simulink model "test"  (R2022b)
settings: Solver=VariableStepAuto  StartTime=0.0  StopTime=300  RelTol=1e-3
values from neighbouring files (symbols this model uses):
  m_pw = zeros(nvw,nwr)    [fun_getwindpowercurve_v4.m]
  pinitwindgen = 0.5161    [WGmodel_startup.m]    (also in WGmodel_startup_v2.m; WGmodel_startup_v3.m = pinitwindgen(1))
  R = 0.05    [WGmodel_startup.m]    (also in WGmodel_startup_v2.m; WGmodel_startup_v3.m)
  Tc2 = 0.05    [WGmodel_startup.m]    (also in WGmodel_startup_v2.m; WGmodel_startup_v3.m)
  v_beta = 0:1:2    [WGmodel_startup.m]    (also in fun_getwindpowercurve_v2.m = 0.5)
  v_pwdel = 0.9 * max(m_pw,[],2)    [fun_getwindpowercurve_v2.m]    (also in fun_getwindpowercurve_v3.m = (1-deload) * v_pwmpp; fun_getwindpowercurve_v4.m = (1-deload) * v_pwmpp)
  v_vw = 5:10    [LUT_2D.m]    (also in WGmodel_startup.m = 5:1:10; WGmodel_startup_v2.m = 5:1:15; WGmodel_startup_v3.m = 5:.5:12; fun_getwindpowercurve_v2.m = [10 11 12])
  v_wr = v_Wr/Wrn    [fun_getwindpowercurve.m]    (also in fun_getwindpowercurve_v2.m; fun_getwindpowercurve_v3.m; fun_getwindpowercurve_v4.m; fun_getwindpowercurve_v5.m)
  v_wrdel = (v_wr(v_iwrmpp+i_lower)+v_wr(v_iwrmpp+i_higher))/2    [fun_getwindpowercurve_v2.m]    (also in fun_getwindpowercurve_v3.m = v_Wrdel/Wrn; fun_getwindpowercurve_v4.m = v_Wrdel/Wrn)
  wr_init = 1.1861    [WGmodel_startup.m]    (also in WGmodel_startup_v2.m)
libraries: slpidlib x2
settings Model: Creator=User  LastModifiedBy=User
settings DataIOCC: ReturnWorkspaceOutputsName=tp07107dd9_9efb_4f85_a9e4_60e1f7b33de8

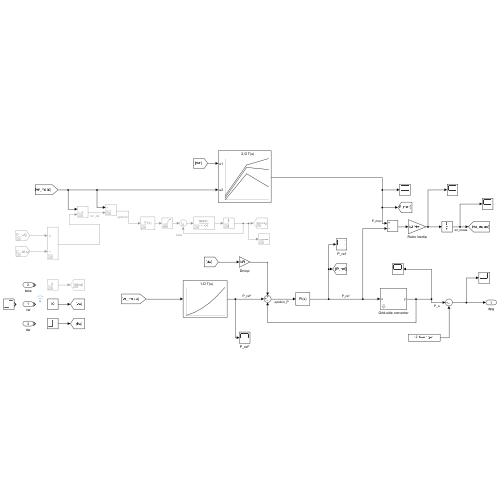
[thumbnail: Simulink's stored preview of the top-level diagram]
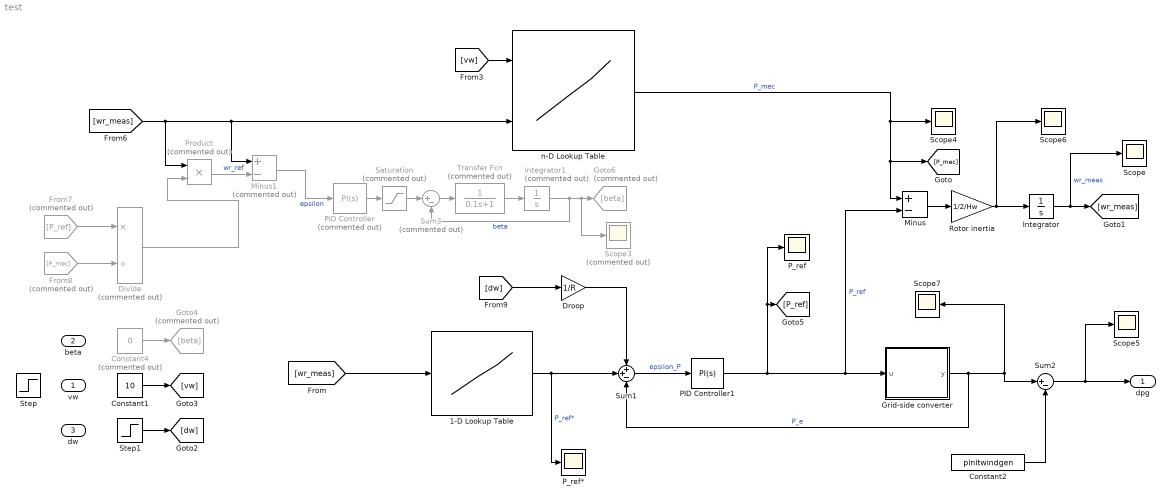
== system test ==
  vw : Inport
  beta : Inport  Port=2
  dw : Inport  Port=3
  1-D Lookup Table : Lookup_n-D  NumberOfTableDimensions=1  BreakpointsForDimension1=v_wrdel  Table=v_pwdel  InternalRulePriority=Speed  RndMeth=Simplest
  Constant1 : Constant  Value=10
  Constant2 : Constant  Value=pinitwindgen
  Constant4 : Constant  Commented=on  Value=0
  Divide : Product  Commented=on  Inputs=*/
  Droop : Gain  Gain=1/R
  From7 : From  Commented=on  GotoTag=P_ref
  From8 : From  Commented=on  GotoTag=P_mec
  Goto4 : Goto  Commented=on  GotoTag=beta
  Goto6 : Goto  Commented=on  GotoTag=beta
  Grid-side converter : Subsystem  mask{T=Tc2, y0=pinitwindgen}
      mask prompts: T "Time constant (s)"; y0 "Initial condition (pu)"
  Integrator : Integrator  InitialCondition=wr_init
  Integrator1 : Integrator  Commented=on
  Minus : Sum  Inputs=+-
  Minus1 : Sum  Commented=on  Inputs=+-
  PID Controller : slpidlib/PID Controller  Commented=on  Controller=PI  Form=Parallel  TimeDomain=Continuous-time  UseExternalTs=off  SampleTime=-1  IntegratorMethod=Forward Euler  FilterMethod=Forward Euler  ControllerParametersSource=internal  P=355  I=0.01  UseKiTs=off  D=0  N=100  UseFilter=on  TunerSelectOption=Transfer Function Based (PID Tuner App)  InitialConditionSource=internal  InitialConditionForIntegrator=0  InitialConditionForFilter=0  DifferentiatorICPrevScaledInput=0  ExternalReset=none  TrackingMode=off  Kt=1  LimitOutput=off  SatLimitsSource=internal  UpperSaturationLimit=inf  LowerSaturationLimit=-inf  LinearizeAsGain=on  AntiWindupMode=none  Kb=1  LimitIntegrator=off  UpperIntegratorSaturationLimit=inf  LowerIntegratorSaturationLimit=-inf  POutMin=[]  POutMax=[]  IOutMin=[]  IOutMax=[]  DOutMin=[]  DOutMax=[]  NOutMin=[]  NOutMax=[]  SumOutMin=[]  SumOutMax=[]  SaturationOutMin=[]  SaturationOutMax=[]  PParamMin=[]  PParamMax=[]  IParamMin=[]  IParamMax=[]  DParamMin=[]  DParamMax=[]  NParamMin=[]  NParamMax=[]  KbParamMin=[]  KbParamMax=[]  KtParamMin=[]  KtParamMax=[]  KbOutMin=[]  KbOutMax=[]  KtOutMin=[]  KtOutMax=[]  IntegratorOutMin=[]  IntegratorOutMax=[]  FilterOutMin=[]  FilterOutMax=[]  SumI1OutMin=[]  SumI1OutMax=[]  SumI2OutMin=[]  SumI2OutMax=[]  SumI3OutMin=[]  SumI3OutMax=[]  SumI4OutMin=[]  SumI4OutMax=[]  SumDOutMin=[]  SumDOutMax=[]  DifferentiatorOutMin=[]  DifferentiatorOutMax=[]  FilterDiffOutCoefMin=[]  FilterDiffOutCoefMax=[]  ReciprocalOutMin=[]  ReciprocalOutMax=[]  SumDenOutMin=[]  SumDenOutMax=[]  SumNumOutMin=[]  SumNumOutMax=[]  DivideOutMin=[]  DivideOutMax=[]  UdiffTsProdOutMin=[]  UdiffTsProdOutMax=[]  NTsProdOutMin=[]  NTsProdOutMax=[]  UintegralTsProdOutMin=[]  UintegralTsProdOutMax=[]  UngainTsProdOutMin=[]  UngainTsProdOutMax=[]  ClampingZeroOutDataTypeStr=Inherit: Inherit via back propagation  ClampingZeroOutMin=[]  ClampingZeroOutMax=[]  FilterDenConstantOutDataTypeStr=Inherit: Inherit via back propagation  FilterDenConstantOutMin=[]  FilterDenConstantOutMax=[]  PCopyOutDataTypeStr=Inherit: Inherit via back propagation  PCopyOutMin=[]  PCopyOutMax=[]  NCopyOutDataTypeStr=Inherit: Inherit via back propagation  NCopyOutMin=[]  NCopyOutMax=[]  IntegratorContinuousStateAttributes=''  IntegratorStateMustResolveToSignalObject=off  IntegratorRTWStateStorageClass=Auto  FilterContinuousStateAttributes=''  FilterStateMustResolveToSignalObject=off  FilterRTWStateStorageClass=Auto  ParallelPVariant=InternalParameters  IdealPVariant=Disabled  IVariant=InternalParameters  DVariant=Disabled  IntegratorVariant=Continuous  SatVariant=Disabled  AWVariant=Passthrough  PCopyVariant=Disabled  TRVariant=Disabled  FdbkBlocksVariant=Forward  IdealPFdbkVariant=Disabled  SatFdbkVariant=Disabled  DerivativeFilterVariant=Disabled  NVariant=Disabled  NCopyVariant=Disabled_SignalSpec  FilterICVariant=Disabled  IntegratorICVariant=InternalICs  ExternalResetVariant=Disabled  TRSumVariant=Passthrough  SumFdbkVariant=Disabled  SumVariant=Sum_PI  TsampFilterVariant=InternalTs  TsampNgainVariant=Passthrough  TsampIntegralVariant=Passthrough  ExternalSaturationOutDataTypeStr=Inherit: Same as second input
  PID Controller1 : slpidlib/PID Controller  Controller=PI  Form=Parallel  TimeDomain=Continuous-time  UseExternalTs=off  SampleTime=-1  IntegratorMethod=Forward Euler  FilterMethod=Forward Euler  ControllerParametersSource=internal  P=1  I=.1  UseKiTs=off  D=0  N=100  UseFilter=on  TunerSelectOption=Transfer Function Based (PID Tuner App)  InitialConditionSource=internal  InitialConditionForIntegrator=Pref_init  InitialConditionForFilter=0  DifferentiatorICPrevScaledInput=0  ExternalReset=none  TrackingMode=off  Kt=1  LimitOutput=off  SatLimitsSource=internal  UpperSaturationLimit=inf  LowerSaturationLimit=-inf  LinearizeAsGain=on  AntiWindupMode=none  Kb=1  LimitIntegrator=off  UpperIntegratorSaturationLimit=inf  LowerIntegratorSaturationLimit=-inf  POutMin=[]  POutMax=[]  IOutMin=[]  IOutMax=[]  DOutMin=[]  DOutMax=[]  NOutMin=[]  NOutMax=[]  SumOutMin=[]  SumOutMax=[]  SaturationOutMin=[]  SaturationOutMax=[]  PParamMin=[]  PParamMax=[]  IParamMin=[]  IParamMax=[]  DParamMin=[]  DParamMax=[]  NParamMin=[]  NParamMax=[]  KbParamMin=[]  KbParamMax=[]  KtParamMin=[]  KtParamMax=[]  KbOutMin=[]  KbOutMax=[]  KtOutMin=[]  KtOutMax=[]  IntegratorOutMin=[]  IntegratorOutMax=[]  FilterOutMin=[]  FilterOutMax=[]  SumI1OutMin=[]  SumI1OutMax=[]  SumI2OutMin=[]  SumI2OutMax=[]  SumI3OutMin=[]  SumI3OutMax=[]  SumI4OutMin=[]  SumI4OutMax=[]  SumDOutMin=[]  SumDOutMax=[]  DifferentiatorOutMin=[]  DifferentiatorOutMax=[]  FilterDiffOutCoefMin=[]  FilterDiffOutCoefMax=[]  ReciprocalOutMin=[]  ReciprocalOutMax=[]  SumDenOutMin=[]  SumDenOutMax=[]  SumNumOutMin=[]  SumNumOutMax=[]  DivideOutMin=[]  DivideOutMax=[]  UdiffTsProdOutMin=[]  UdiffTsProdOutMax=[]  NTsProdOutMin=[]  NTsProdOutMax=[]  UintegralTsProdOutMin=[]  UintegralTsProdOutMax=[]  UngainTsProdOutMin=[]  UngainTsProdOutMax=[]  ClampingZeroOutDataTypeStr=Inherit: Inherit via back propagation  ClampingZeroOutMin=[]  ClampingZeroOutMax=[]  FilterDenConstantOutDataTypeStr=Inherit: Inherit via back propagation  FilterDenConstantOutMin=[]  FilterDenConstantOutMax=[]  PCopyOutDataTypeStr=Inherit: Inherit via back propagation  PCopyOutMin=[]  PCopyOutMax=[]  NCopyOutDataTypeStr=Inherit: Inherit via back propagation  NCopyOutMin=[]  NCopyOutMax=[]  IntegratorContinuousStateAttributes=''  IntegratorStateMustResolveToSignalObject=off  IntegratorRTWStateStorageClass=Auto  FilterContinuousStateAttributes=''  FilterStateMustResolveToSignalObject=off  FilterRTWStateStorageClass=Auto  ParallelPVariant=InternalParameters  IdealPVariant=Disabled  IVariant=InternalParameters  DVariant=Disabled  IntegratorVariant=Continuous  SatVariant=Disabled  AWVariant=Passthrough  PCopyVariant=Disabled  TRVariant=Disabled  FdbkBlocksVariant=Forward  IdealPFdbkVariant=Disabled  SatFdbkVariant=Disabled  DerivativeFilterVariant=Disabled  NVariant=Disabled  NCopyVariant=Disabled_SignalSpec  FilterICVariant=Disabled  IntegratorICVariant=InternalICs  ExternalResetVariant=Disabled  TRSumVariant=Passthrough  SumFdbkVariant=Disabled  SumVariant=Sum_PI  TsampFilterVariant=InternalTs  TsampNgainVariant=Passthrough  TsampIntegralVariant=Passthrough  ExternalSaturationOutDataTypeStr=Inherit: Same as second input
  P_ref : Scope
  P_ref* : Scope
  Product : Product  Commented=on
  Rotor inertia : Gain  Gain=1/2/Hw
  Saturation : Saturate  Commented=on  UpperLimit=10  LowerLimit=-10
  Scope{,4..7} (5 alike) : Scope
  Scope3 : Scope  Commented=on
  Step : Step  Time=10  Before=10  After=12  SampleTime=0
  Step1 : Step  Time=100  After=.001  SampleTime=0
  Sum1 : Sum  Inputs=++-
  Sum2 : Sum  Inputs=|+-
  Sum3 : Sum  Commented=on  Inputs=|+-
  Transfer Fcn : TransferFcn  Commented=on  Denominator=[0.1 1]
  n-D Lookup Table : Lookup_n-D  BreakpointsForDimension1=v_vw  BreakpointsForDimension2=v_wr  BreakpointsForDimension3=v_beta  Table=m_pw  InternalRulePriority=Speed  RndMeth=Simplest
      settings: InputPortMap=u0,u1
  dpg : Outport
  wires:
  Minus/1 -> Rotor inertia/1
  Integrator/1 -> Scope/1, [wr_meas]  "wr_meas"
  Rotor inertia/1 -> Scope6/1, Integrator/1
  n-D Lookup Table/1 -> Minus/1, [P_mec], Scope4/1  "P_mec"
  Sum3/1 -> Transfer Fcn/1
  Saturation/1 -> Sum3/1
  PID Controller/1 -> Saturation/1
  Transfer Fcn/1 -> Integrator1/1
  Integrator1/1 -> Goto6/1, Scope3/1, Sum3/2  "beta"
  From7/1 -> Divide/1
  Divide/1 -> Product/2
  From8/1 -> Divide/2
  PID Controller1/1 -> P_ref/1, [P_ref], Grid-side converter/1(u), Minus/2  "P_ref"
  Droop/1 -> Sum1/1
  [dw] -> Droop/1
  Step1/1 -> [dw]
  Constant1/1 -> [vw]
  Product/1 -> Minus1/2  "wr_ref"
  Constant2/1 -> Sum2/2
  Grid-side converter/1(y) -> Sum1/3, Sum2/1, Scope7/1  "P_e"
  Constant4/1 -> Goto4/1
  [wr_meas] -> Product/1, Minus1/1, n-D Lookup Table/2
  [vw] -> n-D Lookup Table/1
  Minus1/1 -> PID Controller/1  "epsilon"
  [wr_meas] -> 1-D Lookup Table/1
  1-D Lookup Table/1 -> P_ref*/1, Sum1/2  "P_ref*"
  Sum1/1 -> PID Controller1/1  "epsilon_P"
  Sum2/1 -> Scope5/1, dpg/1

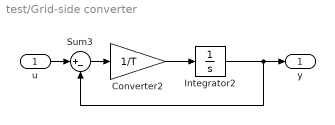
== system test/Grid-side converter ==
  u : Inport
  Converter2 : Gain  Gain=1/T
  Integrator2 : Integrator  InitialCondition=y0
  Sum3 : Sum  Inputs=|+-
  y : Outport
  wires:
  Integrator2/1 -> y/1, Sum3/2
  Sum3/1 -> Converter2/1
  Converter2/1 -> Integrator2/1
  u/1 -> Sum3/1
